simulink model "SimulinkModel_hquad_lin_thrust_0thOrd"  (Simulink 7.6)
settings: Solver=ode45  StartTime=0.0  StopTime=10.0  RelTol=1e-3
values from neighbouring files (symbols this model uses):
  mass = 0.66    [kostas_malakies.mat]    (also in kostas_malakies2.mat; load_PMModel.m = 0.687; main_last.m)
libraries: Hqaud_model_LIB_SI x1
settings Model: Creator=andi  LastModifiedBy=burrimi
settings DebuggingCC: StrictBusMsg=Warning

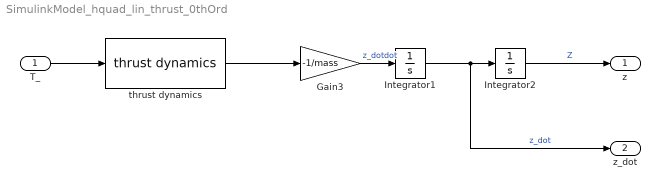
== system SimulinkModel_hquad_lin_thrust_0thOrd ==
  "T_  " : Inport
  Gain3 : Gain  Gain=-1/mass
  Integrator1 : Integrator
  Integrator2 : Integrator
  "thrust dynamics  " : Hqaud_model_LIB_SI/thrust dynamics    SystemSampleTime=-1
  "z " : Outport
  z_dot : Outport  Port=2
  wires:
  "T_  "/1 -> "thrust dynamics  "/1
  Integrator2/1 -> "z "/1  "Z"
  Integrator1/1 -> Integrator2/1, z_dot/1  "z_dot"
  Gain3/1 -> Integrator1/1  "z_dotdot"
  "thrust dynamics  "/1 -> Gain3/1
